simulink model "ModeAdjust"  (R2018b)
settings: Solver=FixedStepDiscrete  StartTime=0.0  StopTime=inf  FixedStep=0.01  RelTol=1e-3
undefined symbols (not defined in the file or in its folder): IfKeSMSbSeatMovBkRclnEnable_Val, IfKeSMSbSeatMovFrwdBkwdEnable_Val, IfKeSMSbSeatMovFtrstEnable_Val, IfKeSMSbSeatMovHdrstFrwdBkwdEnable_Val, IfKeSMSbSeatMovHdUpwdDnwdEnable_Val, IfKeSMSbSeatMovLgrstEnable_Val, IfKeSMSbSeatMovLtwdRtwdEnable_Val, IfVeSMSeStNumConfig, KeSMSbArmscreenMovEnable_Val, KeSMSbSeatMovLgrstExpdEnable_Val, KeSMSuFirstRwStBackPosDelta_Val, KeSMSuFirstRwStBackPosTolr_Val, KeSMSuFirstRwStCushFrntPosDelta_Val, KeSMSuFirstRwStCushFrntPosTolr_Val, KeSMSuFirstRwStCushRePosDelta_Val, KeSMSuFirstRwStCushRePosTolr_Val, KeSMSuFirstRwStFootrestPosDelta_Val, KeSMSuFirstRwStFootrestPosTolr_Val, KeSMSuFirstRwStFwdBkwdPosDelta_Val, KeSMSuFirstRwStFwdBkwdPosTolr_Val, KeSMSuMdMotFinshdTm_Val, KeSMSuMdRetryTm1_Val, KeSMSuModeReqDurgTm_Val, KeSMSuSecRwStArmTochPosDelta_Val, KeSMSuSecRwStArmTochPosTolr_Val, KeSMSuSecRwStBackPosDelta_Val, KeSMSuSecRwStBackPosTolr_Val, KeSMSuSecRwStFtrstUpwdDnwdPosDelta_Val, KeSMSuSecRwStFtrstUpwdDnwdPosTolr_Val, KeSMSuSecRwStFwdBkwdPosDelta_Val, KeSMSuSecRwStFwdBkwdPosTolr_Val, KeSMSuSecRwStHeadrestFwdBkwdPosDelta_Val, KeSMSuSecRwStHeadrestFwdBkwdPosTolr_Val, KeSMSuSecRwStHeadrestUpwdDwnwdPosDelta_Val, KeSMSuSecRwStHeadrestUpwdDwnwdPosTolr_Val, KeSMSuSecRwStLegrestInOutPosDelta_Val, KeSMSuSecRwStLegrestInOutPosTolr_Val, KeSMSuSecRwStLegrestUpwdDwnwdPosDelta_Val, KeSMSuSecRwStLegrestUpwdDwnwdPosTolr_Val, KeSMSuSecRwStLwdRwdPosDelta_Val, KeSMSuSecRwStLwdRwdPosTolr_Val, KeSMSuSecRwStVIPFtrstRefAngle_Val, KeSMSuThirdRwStFwdBkwdPosDelta_Val, KeSMSuThirdRwStFwdBkwdPosTolr_Val, KeSMSuThrdRwCushFoldPosDelta_Val, KeSMSuThrdRwCushFoldPosTolr_Val, KeSMSuThrdRwStBackPosDelta_Val, KeSMSuThrdRwStBackPosTolr_Val, KeSMSw4SLegrstCloseMdSecRwLtStFtrstUpwdDnwdPos_Val, KeSMSw4SLegrstCloseMdSecRwLtStFtrstUpwdDnwdPosMax_Val, KeSMSw4SLegrstCloseMdSecRwLtStFtrstUpwdDnwdPosMin_Val, KeSMSw4SLegrstCloseMdSecRwLtStLgrstOtwdInwdPos_Val, KeSMSw4SLegrstCloseMdSecRwLtStLgrstOtwdInwdPosMax_Val, KeSMSw4SLegrstCloseMdSecRwLtStLgrstOtwdInwdPosMin_Val, KeSMSw4SLegrstCloseMdSecRwLtStLgrstUpwdDnwdPos_Val, KeSMSw4SLegrstCloseMdSecRwLtStLgrstUpwdDnwdPosMax_Val, KeSMSw4SLegrstCloseMdSecRwLtStLgrstUpwdDnwdPosMin_Val, KeSMSw4SLegrstCloseMdSecRwRtStFtrstUpwdDnwdPos_Val, KeSMSw4SLegrstCloseMdSecRwRtStFtrstUpwdDnwdPosMax_Val, KeSMSw4SLegrstCloseMdSecRwRtStFtrstUpwdDnwdPosMin_Val ... (+1138)
libraries: Lib x401
(part 10 of 35)

== system ModeAdjust/ModeAdjustRunnable_sys/ModeAdjust/RecvyR4s ==
  note: Change Request 179276
      | 复位模式头枕上下移动到第一步，第一步直接控制靠背、头枕上下、腿托系统同时运动，
      | 当腿托系统运动完成后进行头枕前后运动
  SecRwLtStsPoss : Inport
  SecRwLtStPossV : Inport  Port=2
  SecRwRtStChldLkRsp_L : Inport  Port=3
  Recovery_Mod_Left : Inport  Port=4
  ModeStCalib : Inport  Port=5
  StConfig : Inport  Port=6
  SecRwLtStsPoss4s : Inport  Port=7
  SecRwLtStPossV4s : Inport  Port=8
  StConfig4s : Inport  Port=9
  isRtRecoveryArrivedAtTargetPos : Inport  Port=10
  Calib_Recovery4sRAdpt : Inport  Port=11
  Enable : EnablePort  StatesWhenEnabling=reset
  Bus Creator1 : BusCreator  Inputs=2
  Bus Selector : BusSelector  OutputSignals=Calib_Drv,Calib_Pass,Calib_2L,Calib_2R,Calib_3L,Calib_3R,Calib_2L4s,Calib_2R4s
  Bus Selector1 : BusSelector  OutputSignals=DrvStConfig,PassStConfig,SecRwLtStConfig,SecRwRtStConfig,ThdRwLtStConfig,ThdRwRtStConfig
  Bus Selector2 : BusSelector  OutputSignals=SecRwLtStConfig,SecRwRtStConfig
  Bus Selector3 : BusSelector  OutputSignals=IfVeSMSuSecRwRtStBkReclnUpwdDnwdPos_Val_read,IfVeSMSuSecRwRtStFrwdBkwdPos_Val_read,IfVeSMSuSecRwRtStHPassStUpwdDnwdPos_Val_read,IfVeSMSuSecRwRtStLgrstUpwdDnwdPos_Val_read,IfVeSMSuSecRwRtStLtwdRtwdPos_Val_read,SecRwRtStArmScrnPos_Val_read
  Bus Selector4 : BusSelector  OutputSignals=IfVeSMSuSecRwRtStBkReclnUpwdDnwdPosV_Val_read,IfVeSMSuSecRwRtStFrwdBkwdPosV_Val_read,IfVeSMSuSecRwRtStHPassStUpwdDnwdPosV_Val_read,IfVeSMSuSecRwRtStLgrstUpwdDnwdPosV_Val_read,IfVeSMSuSecRwRtStLtwdRtwdPosV_Val_read,SecRwRtStArmScrnPosV_Val_read
  Bus Selector5 : BusSelector  OutputSignals=IfVeSMSuSecRwRtStLgrstOtwdInwdPos_Val_read,IfVeSMSuRrRtStFtUpwdDnwdPos_Val_read,IfVeSMSuSecRwRtStHdrstFrwdBkwdPos_Val_read
  Bus Selector6 : BusSelector  OutputSignals=IfVeSMSuSecRwRtStLgrstOtwdInwdPosV_Val_read,IfVeSMSuRrRtStFtUpwdDnwdPosV_Val_read
  Chart : Stateflow chart  TreatAsAtomicUnit=on
  Chart1 : Stateflow chart  TreatAsAtomicUnit=on
  Logical Operator : Logic  Inputs=4  AllPortsSameDT=off  OutDataTypeStr=boolean
  Logical Operator1 : Logic  Operator=NOT  AllPortsSameDT=off  OutDataTypeStr=boolean
  Logical Operator2 : Logic  Inputs=3  AllPortsSameDT=off  OutDataTypeStr=boolean
  Logical Operator3 : Logic  Operator=OR  AllPortsSameDT=off  OutDataTypeStr=boolean
  PA_KeSMSuSecRwStFtrstUpwdDnwdPosDelta_Val : Constant  Value=KeSMSuSecRwStFtrstUpwdDnwdPosDelta_Val
  PA_KeSMSuSecRwStLegrestInOutPosDelta_Val : Constant  Value=KeSMSuSecRwStLegrestInOutPosDelta_Val
  PA_KeSMSw4SSecRwRtStLgrstOtwdInwdClosePos1_Val : Constant  Value=KeSMSw4SSecRwRtStLgrstOtwdInwdClosePos1_Val
  PA_KeSMSw4SSecRwRtStLgrstUpwdDnwdClosePos1_Val : Constant  Value=KeSMSw4SSecRwRtStLgrstUpwdDnwdClosePos1_Val
  PA_KeSMSw4SSecRwRtStLgrstUpwdDnwdClosePos2_Val : Constant  Value=KeSMSw4SSecRwRtStLgrstUpwdDnwdClosePos2_Val
  R2Lt : Subsystem
  VIP_TrigJudg : Lib/VIP_TrigJudg  SystemSampleTime=-1
  R2Lt_TrgtPoss : Outport  VectorParamsAs1DForOutWhenUnconnected=on
  IfVeSMSuSecRwLtStRclCmdSrv_Val_writeRec : Outport  Port=2
  isAcsMdFeedBackNew_LyL : Outport  Port=3
  R2Lt_TrgtPoss_2 : Outport  Port=4  VectorParamsAs1DForOutWhenUnconnected=on
  wires:
  R2Lt/6(lgrstFtUpwd_ini) -> [lgrstStep3_ini]
  R2Lt/7(lgrstOtwd_ini) -> [lgrstStep1_ini]
  R2Lt/5(lgrstUpwd_ini) -> [lgrstStep2_ini]
  R2Lt/9(lgrstStep2_done) -> [lgrstStep3_done]
  R2Lt/10(lgrstStep3_done) -> [lgrstStep1_done]
  R2Lt/8(lgrstStep1_done) -> [lgrstStep2_done]
  [KeSMSuSecRwStFtrstUpwdDnwdPosDelta_Val] -> Chart/15(FtposDelta)
  PA_KeSMSuSecRwStFtrstUpwdDnwdPosDelta_Val/1 -> [KeSMSuSecRwStFtrstUpwdDnwdPosDelta_Val]
  [StepEn_LgrstStep2] -> R2Lt/11(StepEn_LgrstStep1)
  [StepEn_LgrstStep3] -> R2Lt/12(StepEn_LgrstStep2)
  [StepEn_LgrstStep1] -> R2Lt/13(StepEn_LgrstStep3)
  [SecRwLtStLgrstOtwdInwdPos] -> Chart/4(Otpos)
  [RrLtStFtUpwdDnwdPos] -> Chart/5(Ftpos)
  [CloseOtwdPos1] -> Chart/8(closeOtpos1)
  [CloseDnwdPos1] -> Chart/6(closedownpos1)
  [CloseDnwdPos2] -> Chart/7(closedownpos2)
  PA_KeSMSw4SSecRwRtStLgrstUpwdDnwdClosePos1_Val/1 -> [CloseDnwdPos1]
  PA_KeSMSw4SSecRwRtStLgrstUpwdDnwdClosePos2_Val/1 -> [CloseDnwdPos2]
  PA_KeSMSw4SSecRwRtStLgrstOtwdInwdClosePos1_Val/1 -> [CloseOtwdPos1]
  [lgrstStep3_done] -> Chart/11(Step3done)
  R2Lt/11(R2Lt_TrgtPoss_2) -> R2Lt_TrgtPoss_2/1
  Chart/4(StepEn_LgrstStep3) -> [StepEn_LgrstStep3]
  Chart/3(StepEn_LgrstStep2) -> [StepEn_LgrstStep2]
  Chart/2(StepEn_LgrstStep1) -> [StepEn_LgrstStep1]
  [lgrstStep2_done] -> Chart/10(Step2done)
  [lgrstStep3_ini] -> Chart/14(Step3_ini)
  [lgrstStep2_ini] -> Chart/13(Step2_ini)
  [lgrstStep1_ini] -> Chart/12(Step1_ini)
  [lgrstStep1_done] -> Chart/9(Step1done)
  [SecRwLtStLgrstUpwdDnwdPos] -> Chart/3(downpos)
  Bus Selector5/2 -> [RrLtStFtUpwdDnwdPos]  "<IfVeSMSuRrRtStFtUpwdDnwdPos_Val_read>"
  Bus Selector5/1 -> [SecRwLtStLgrstOtwdInwdPos]  "<IfVeSMSuSecRwRtStLgrstOtwdInwdPos_Val_read>"
  [PosV4s] -> Bus Selector6/1
  Bus Selector6/2 -> [RrLtStFtUpwdDnwdPosV]  "<IfVeSMSuRrRtStFtUpwdDnwdPosV_Val_read>"
  [Pos4s] -> Bus Selector5/1
  Bus Selector6/1 -> [SecRwLtStLgrstOtwdInwdPosV]  "<IfVeSMSuSecRwRtStLgrstOtwdInwdPosV_Val_read>"
  Bus Selector4/1 -> [SecRwLtStBkReclnUpwdDnwdPosV]  "<IfVeSMSuSecRwRtStBkReclnUpwdDnwdPosV_Val_read>"
  Bus Selector4/3 -> [SecRwLtStHPassStUpwdDnwdPosV]  "<IfVeSMSuSecRwRtStHPassStUpwdDnwdPosV_Val_read>"
  Bus Selector3/5 -> [SecRwLtStLtwdRtwdPos]  "<IfVeSMSuSecRwRtStLtwdRtwdPos_Val_read>"
  [Pos] -> Bus Selector3/1
  Bus Selector3/3 -> [SecRwLtStHPassStUpwdDnwdPos]  "<IfVeSMSuSecRwRtStHPassStUpwdDnwdPos_Val_read>"
  Bus Selector4/4 -> [SecRwLtStLgrstUpwdDnwdPosV]  "<IfVeSMSuSecRwRtStLgrstUpwdDnwdPosV_Val_read>"
  Bus Selector4/2 -> [SecRwLtStFrwdBkwdPosV]  "<IfVeSMSuSecRwRtStFrwdBkwdPosV_Val_read>"
  Bus Selector3/2 -> [SecRwLtStFrwdBkwdPos]  "<IfVeSMSuSecRwRtStFrwdBkwdPos_Val_read>"
  Bus Selector3/1 -> [SecRwLtStBkReclnUpwdDnwdPos]  "<IfVeSMSuSecRwRtStBkReclnUpwdDnwdPos_Val_read>"
  Bus Selector3/4 -> [SecRwLtStLgrstUpwdDnwdPos]  "<IfVeSMSuSecRwRtStLgrstUpwdDnwdPos_Val_read>"
  Bus Selector4/5 -> [SecRwLtStLtwdRtwdPosV]  "<IfVeSMSuSecRwRtStLtwdRtwdPosV_Val_read>"
  Bus Selector3/6 -> [R2LtStArmScrnPos]  "<SecRwRtStArmScrnPos_Val_read>"
  Bus Selector4/6 -> [R2LtStArmScrnPosV]  "<SecRwRtStArmScrnPosV_Val_read>"
  [PosV] -> Bus Selector4/1
  [SecRwLtStConfig4s] -> R2Lt/10(StConfig4s)
  Bus Selector2/2 -> [SecRwRtStConfig4s]  "<SecRwRtStConfig>"
  Bus Selector2/1 -> [SecRwLtStConfig4s]  "<SecRwLtStConfig>"
  StConfig4s/1 -> Bus Selector2/1
  SecRwLtStPossV4s/1 -> R2Lt/9(SecRwLtStPossV4s), [PosV4s]
  SecRwLtStsPoss4s/1 -> [Pos4s], R2Lt/8(SecRwLtStsPoss4s)
  Bus Selector/7 -> [ModeStCalib_2L4s]  "<Calib_2L4s>"
  Bus Selector/8 -> [ModeStCalib_2R4s]  "<Calib_2R4s>"
  [SecRwLtStConfig] -> R2Lt/7(StConfig)
  Bus Selector1/5 -> [ThdRwLtStConfig]  "<ThdRwLtStConfig>"
  Bus Selector1/2 -> [PassStConfig]  "<PassStConfig>"
  StConfig/1 -> Bus Selector1/1
  Bus Selector1/4 -> [SecRwRtStConfig]  "<SecRwRtStConfig>"
  Bus Selector1/3 -> [SecRwLtStConfig]  "<SecRwLtStConfig>"
  Bus Selector1/1 -> [DrvStConfig]  "<DrvStConfig>"
  Bus Selector1/6 -> [ThdRwRtStConfig]  "<ThdRwRtStConfig>"
  [Ly_L_DoneFailed] -> Bus Creator1/2  "isRfRecoveryDoneFailed"
  [Ly_L_DoneOK] -> Bus Creator1/1  "isRfRecoveryDoneOK"
  Bus Creator1/1 -> isAcsMdFeedBackNew_LyL/1
  [Recovery_Mod_Left] -> VIP_TrigJudg/1
  [ModeStCalib_2R4s] -> R2Lt/6(ModeStCalib_2L)
  ModeStCalib/1 -> Bus Selector/1
  Bus Selector/4 -> [ModeStCalib_2R]  "<Calib_2R>"
  Bus Selector/6 -> [ModeStCalib_3R]  "<Calib_3R>"
  Bus Selector/1 -> [ModeStCalib_Drv]  "<Calib_Drv>"
  Bus Selector/3 -> [ModeStCalib_2L]  "<Calib_2L>"
  Bus Selector/5 -> [ModeStCalib_3L]  "<Calib_3L>"
  Bus Selector/2 -> [ModeStCalib_Pass]  "<Calib_Pass>"
  Chart1/1(IfVeSMSuSecRwLtStRclCmdSrv_Val_write) -> IfVeSMSuSecRwLtStRclCmdSrv_Val_writeRec/1  "IfVeSMSuSecRwLtStRclCmdSrv_Val_write"
  Chart1/3(Md_L_DoneFailed) -> [Ly_L_DoneFailed]
  Chart1/2(Md_L_DoneOk) -> [Ly_L_DoneOK]
  [Recv_L_DoneFailed] -> Chart1/4(Md_L_DoneFailedRaw)
  [Recv_L_DoneOK] -> Chart1/3(Md_L_DoneOkRaw)
  Chart/1(R2Lt_En) -> [Step1_En]
  [R2LtST_BkHd_done] -> Chart/2(R2Lt_done)
  [R2LtST_BkHd_ini] -> Chart/1(R2Lt_ini)
  R2Lt/2(R2Lt_BkHd_done) -> [R2LtST_BkHd_done]
  SecRwRtStChldLkRsp_L/1 -> R2Lt/5(SecRwRtStChldLkRsp_L)
  SecRwLtStPossV/1 -> [PosV], R2Lt/4(SecRwLtStPossV)
  SecRwLtStsPoss/1 -> [Pos], R2Lt/3(SecRwLtStsPoss)
  R2Lt/3(R2Lt_TrgtPoss) -> R2Lt_TrgtPoss/1
  [EZE_TrigL] -> R2Lt/1(Mode_Trig)
  VIP_TrigJudg/1 -> [EZE_TrigL]
  [Step1_En] -> R2Lt/2(Step1En)
  R2Lt/1(R2Lt_BkHd_Ini) -> [R2LtST_BkHd_ini]
  Logical Operator/1 -> Chart1/1(Left_Done)
  Recovery_Mod_Left/1 -> [Recovery_Mod_Left]
  [IfVeSMSuSecRwLtStRclCmdSrv_Val_writeRaw] -> Chart1/2(IfVeSMSuSecRwLtStRclCmdSrv_Val_writeRaw)
  R2Lt/4(IfVeSMSuSecRwLtStRclCmdSrv_Val_writeRaw) -> [IfVeSMSuSecRwLtStRclCmdSrv_Val_writeRaw]
  Logical Operator1/1 -> [Recv_L_DoneFailed]
  isRtRecoveryArrivedAtTargetPos/1 -> [Recv_L_DoneOK], Logical Operator1/1
  Chart/5(HdUp_En) -> [HdUp_En]
  Chart/6(HdFwd_En) -> [HdFwd_En]
  [HdUp_Done] -> Chart/17(HdUp_Done)
  [HFwd_Done] -> Chart/16(HdFwd_Done)
  Bus Selector5/3 -> [SecRwLtStHdrstFrwdBkwdPos]  "<IfVeSMSuSecRwRtStHdrstFrwdBkwdPos_Val_read>"
  R2Lt/14(R2Lt_HdFwd_Ini) -> [HFwd_ini]
  R2Lt/12(R2Lt_HdUp_Ini) -> [HdUp_ini]
  R2Lt/15(R2Lt_HdFwd_Done) -> [HFwd_Done]
  R2Lt/13(R2Lt_HdUp_Done) -> [HdUp_Done]
  [HdUp_En] -> R2Lt/14(HdUp_En)
  [HdFwd_En] -> R2Lt/15(HdFwd_En)
  PA_KeSMSuSecRwStLegrestInOutPosDelta_Val/1 -> [KeSMSuSecRwStLegrestInOutPosDelta_Val]
  [KeSMSuSecRwStLegrestInOutPosDelta_Val] -> Chart/18(OtposDelta)
  Chart/7(failflg) -> [failflg]
  [lgrstStep1_done] -> Logical Operator2/1
  [lgrstStep2_done] -> Logical Operator2/2
  [lgrstStep3_done] -> Logical Operator2/3
  Logical Operator2/1 -> Logical Operator3/2
  [failflg] -> Logical Operator3/1
  Logical Operator3/1 -> Logical Operator/1
  [HdUp_Done] -> Logical Operator/4
  [HFwd_Done] -> Logical Operator/3
  [R2LtST_BkHd_done] -> Logical Operator/2
  [HdUp_ini] -> Chart/19(HdUp_ini)
  [HFwd_ini] -> Chart/20(HFwd_ini)
  Calib_Recovery4sRAdpt/1 -> R2Lt/16(Calib_Recovery4sRAdpt)

== system ModeAdjust/ModeAdjustRunnable_sys/ModeAdjust/SeatOccupyCheck ==
  IfVeSMSeNotThdRwCtStOccStatMSMSrc_Val_read : Inport
  IfVeSMSeNotThdRwLtStOccStatMSMSrc_Val_read : Inport  Port=2
  IfVeSMSeNotThdRwRtStOccStatMSMSrc_Val_read : Inport  Port=3
  StNumConfig : Inport  Port=4
  Bus Creator : BusCreator  Inputs=3
  Bus Creator1 : BusCreator  Inputs=3
  Bus Creator2 : BusCreator  Inputs=3
  Bus Selector : BusSelector  OutputSignals=LtStOccStat,CtStOccStat,RtStOccStat
  Constant{,1..3} (4 alike) : Constant  Value=SeatOccupiedSts1.SeatOccupiedSts_Empty  OutDataTypeStr=Enum:SeatOccupiedSts1
  Multiport Switch4 : MultiPortSwitch  DataPortOrder=Specify indices  DataPortIndices={IfVeSMSeStNumConfig.SeatNum4Config,IfVeSMSeStNumConfig.SeatNum6Config,IfVeSMSeStNumConfig.SeatNum7Config,IfVeSMSeStNumConfig.SeatNum4PConfig}  DataPortForDefault=Additional data port  DiagnosticForDefault=None
  SeatOccupiedStat : Lib/SeatOccupiedStat  SystemSampleTime=-1
  SeatOccupiedStat1 : Lib/SeatOccupiedStat  SystemSampleTime=-1
  SeatOccupiedStat2 : Lib/SeatOccupiedStat  SystemSampleTime=-1
  isR3LfSeatOccupied : Outport
  isR3MidSeatOccupied : Outport  Port=2
  isR3RtSeatOccupied : Outport  Port=3
  wires:
  SeatOccupiedStat/1 -> isR3LfSeatOccupied/1  "isR3LfSeatOccupied"
  SeatOccupiedStat1/1 -> isR3MidSeatOccupied/1  "isR3MidSeatOccupied"
  SeatOccupiedStat2/1 -> isR3RtSeatOccupied/1  "isR3RtSeatOccupied"
  StNumConfig/1 -> Multiport Switch4/1
  IfVeSMSeNotThdRwCtStOccStatMSMSrc_Val_read/1 -> Bus Creator/2  "CtStOccStat"
  Bus Creator/1 -> Multiport Switch4/6, Multiport Switch4/4
  Multiport Switch4/1 -> Bus Selector/1
  Constant2/1 -> Bus Creator1/3  "RtStOccStat"
  Constant/1 -> Bus Creator1/1  "LtStOccStat"
  Bus Creator1/1 -> Multiport Switch4/2, Multiport Switch4/5
  Constant1/1 -> Bus Creator1/2  "CtStOccStat"
  Constant3/1 -> Bus Creator2/2  "CtStOccStat"
  Bus Creator2/1 -> Multiport Switch4/3
  IfVeSMSeNotThdRwLtStOccStatMSMSrc_Val_read/1 -> Bus Creator/1, Bus Creator2/1  "LtStOccStat"
  IfVeSMSeNotThdRwRtStOccStatMSMSrc_Val_read/1 -> Bus Creator2/3, Bus Creator/3  "RtStOccStat"
  Bus Selector/1 -> SeatOccupiedStat/1  "<LtStOccStat>"
  Bus Selector/2 -> SeatOccupiedStat1/1  "<CtStOccStat>"
  Bus Selector/3 -> SeatOccupiedStat2/1  "<RtStOccStat>"

== system ModeAdjust/ModeAdjustRunnable_sys/ModeAdjust/SecRowSeatOccupyCheck ==
  IfVeSMSeNotSecRowLeSeaOccStat_Val_read : Inport
  IfVeSMSeNotSecRowRtSeaOccStat_Val_read : Inport  Port=2
  SeatOccupiedStat : Lib/SeatOccupiedStat  SystemSampleTime=-1
  SeatOccupiedStat1 : Lib/SeatOccupiedStat  SystemSampleTime=-1
  isSecRowLtSeatOccupied : Outport  VectorParamsAs1DForOutWhenUnconnected=on
  isSecRowRtSeatOccupied : Outport  Port=2  VectorParamsAs1DForOutWhenUnconnected=on
  wires:
  IfVeSMSeNotSecRowLeSeaOccStat_Val_read/1 -> SeatOccupiedStat/1
  IfVeSMSeNotSecRowRtSeaOccStat_Val_read/1 -> SeatOccupiedStat1/1
  SeatOccupiedStat/1 -> isSecRowLtSeatOccupied/1  "isSecRowLtSeatOccupied"
  SeatOccupiedStat1/1 -> isSecRowRtSeatOccupied/1  "isSecRowRtSeatOccupied"

== system ModeAdjust/ModeAdjustRunnable_sys/ModeAdjust/Subsystem ==
  StNumConfig : Inport
  Logical Operator1 : Logic  Operator=OR  AllPortsSameDT=off  OutDataTypeStr=boolean
  Logical Operator9 : Logic  Operator=OR  AllPortsSameDT=off  OutDataTypeStr=boolean
  PA_KeSMSwDltTrgtPos_Val1 : Constant  Value=IfVeSMSeStNumConfig.SeatNum6Config  OutDataTypeStr=Enum:IfVeSMSeStNumConfig
  PA_KeSMSwDltTrgtPos_Val10 : Constant  Value=IfVeSMSeStNumConfig.SeatNum7Config  OutDataTypeStr=Enum:IfVeSMSeStNumConfig
  PA_KeSMSwDltTrgtPos_Val2 : Constant  Value=IfVeSMSeStNumConfig.SeatNum4Config  OutDataTypeStr=Enum:IfVeSMSeStNumConfig
  PA_KeSMSwDltTrgtPos_Val3 : Constant  Value=IfVeSMSeStNumConfig.SeatNum4PConfig  OutDataTypeStr=Enum:IfVeSMSeStNumConfig
  Relational Operator{1..3,10} (4 alike) : RelationalOperator  Operator===  OutDataTypeStr=boolean  RndMeth=Simplest
  is6s7s : Outport
  is4s : Outport  Port=2
  is6s : Outport  Port=3
  is7s : Outport  Port=4
  wires:
  Relational Operator1/1 -> is6s/1, Logical Operator9/1  "is6s"
  Logical Operator9/1 -> is6s7s/1  "is6s7s"
  [StNumConfig] -> Relational Operator1/1
  [StNumConfig] -> Relational Operator10/1
  PA_KeSMSwDltTrgtPos_Val1/1 -> Relational Operator1/2
  Relational Operator10/1 -> is7s/1, Logical Operator9/2  "is7s"
  PA_KeSMSwDltTrgtPos_Val10/1 -> Relational Operator10/2
  StNumConfig/1 -> [StNumConfig]
  [StNumConfig] -> Relational Operator2/1
  PA_KeSMSwDltTrgtPos_Val2/1 -> Relational Operator2/2
  [StNumConfig] -> Relational Operator3/1
  PA_KeSMSwDltTrgtPos_Val3/1 -> Relational Operator3/2
  Relational Operator2/1 -> Logical Operator1/1
  Relational Operator3/1 -> Logical Operator1/2
  Logical Operator1/1 -> is4s/1  "is4s"

== system ModeAdjust/ModeAdjustRunnable_sys/ModeAdjust/VIPL ==
  SecRwLtStsPoss : Inport
  SecRwLtStPossV : Inport  Port=2
  ThdRwLtStPoss : Inport  Port=3
  ThdRwLtStPossV : Inport  Port=4
  SecRwRtStChldLkRsp_L : Inport  Port=5
  isR3MidSeatOccupied : Inport  Port=6
  isR3LfSeatOccupied : Inport  Port=7
  VIP_Mod_Left : Inport  Port=8
  ModeStCalib : Inport  Port=9
  StConfig : Inport  Port=10
  DrvCurPos : Inport  Port=11
  DrvCurPosV : Inport  Port=12
  isLfVipArrivedAtTargetPos : Inport  Port=13
  Drv_FtUpwdDnwdPosTrgt : Inport  Port=14
  Enable : EnablePort  StatesWhenEnabling=reset
  Bus Creator1 : BusCreator  Inputs=2
  Bus Selector : BusSelector  OutputSignals=Calib_Drv,Calib_Pass,Calib_2L,Calib_2R,Calib_3L,Calib_3R
  Bus Selector1 : BusSelector  OutputSignals=DrvStConfig,PassStConfig,SecRwLtStConfig,SecRwRtStConfig,ThdRwLtStConfig,ThdRwRtStConfig
  Chart1 : Stateflow chart  TreatAsAtomicUnit=on
  Chart2 : Stateflow chart  TreatAsAtomicUnit=on
  Drv : Subsystem
  Logical Operator{,5,9,12} (4 alike) : Logic  Inputs=3  AllPortsSameDT=off  OutDataTypeStr=boolean
  Logical Operator{1,11,14..15} (4 alike) : Logic  AllPortsSameDT=off  OutDataTypeStr=boolean
  Logical Operator{4,6..7,13} (4 alike) : Logic  Operator=OR  AllPortsSameDT=off  OutDataTypeStr=boolean
  Logical Operator2 : Logic  Operator=NOT  AllPortsSameDT=off  OutDataTypeStr=boolean
  R2Lt : Subsystem
  R3Lt : Subsystem
  Terminator3 : Terminator
  Unit Delay1 : UnitDelay  SampleTime=-1
  Unit Delay3 : UnitDelay  SampleTime=-1
  Unit Delay4 : UnitDelay  SampleTime=-1
  VIP_TrigJudg : Lib/VIP_TrigJudg  SystemSampleTime=-1
  R2Lt_TrgtPoss : Outport  VectorParamsAs1DForOutWhenUnconnected=on
  R3Lt_TrgtPoss : Outport  Port=2  VectorParamsAs1DForOutWhenUnconnected=on
  IfVeSMSbThdRwLtStRclCmdSrv_Val_writeVIP : Outport  Port=3
  IfVeSMSuSecRwLtStRclCmdSrv_Val_writeVIP : Outport  Port=4
  isAcsMdFeedBackNew_VIPL : Outport  Port=5
  VIPLDone : Outport  Port=6
  DrvStTrgtPoss : Outport  Port=7  VectorParamsAs1DForOutWhenUnconnected=on
  IfVeSMSuDrvStRclCmdSrv_Val_write : Outport  Port=8
  R2Lt_SpdCtrl : Outport  Port=9  VectorParamsAs1DForOutWhenUnconnected=on
  R3Lt_SpdCtrl : Outport  Port=10  VectorParamsAs1DForOutWhenUnconnected=on
  wires:
  isR3MidSeatOccupied/1 -> Logical Operator4/1
  SecRwRtStChldLkRsp_L/1 -> [SecRwRtStChldLkRsp_L], R2Lt/7(SecRwRtStChldLkRsp_L)
  ThdRwLtStPossV/1 -> R3Lt/5(ThdRwLtStPossV)
  ThdRwLtStPoss/1 -> R3Lt/4(ThdRwLtStPoss)
  SecRwLtStPossV/1 -> R2Lt/6(SecRwLtStPossV)
  SecRwLtStsPoss/1 -> R2Lt/5(SecRwLtStsPoss)
  [EZE_TrigL] -> R3Lt/1(Mode_Trig)
  R3Lt/4(R3Lt_TrgtPoss) -> R3Lt_TrgtPoss/1
  R2Lt/7(R2Lt_TrgtPoss) -> R2Lt_TrgtPoss/1
  [EZE_TrigL] -> R2Lt/1(Mode_Trig)
  [IfVeSMSbThdRwLtStRclCmdSrv_Val_writeRaw] -> Chart1/2(IfVeSMSbThdRwLtStRclCmdSrv_Val_writeRaw)
  R3Lt/3(IfVeSMSbThdRwLtStRclCmdSrv_Val_writeRaw) -> [IfVeSMSbThdRwLtStRclCmdSrv_Val_writeRaw]
  R2Lt/6(R2Lt_Step2_done) -> [R2LtST_Step2_done]  "VIPL_R2LtST_Step2_done"
  R2Lt/5(R2Lt_Step1_done) -> [R2LtST_Step1_done]  "VIPL_R2LtST_Step1_done"
  R2Lt/4(R2Lt_Step2_Ini) -> [R2LtST_Step2_ini]
  R2Lt/1(R2Lt_Step1_Ini) -> [R2LtST_Step1_ini]
  R3Lt/1(R3Lt_Step1_ini) -> [R3Lt_Step1_ini]
  Logical Operator4/1 -> [Occupied]
  isR3LfSeatOccupied/1 -> Logical Operator4/2
  VIP_TrigJudg/1 -> [EZE_TrigL]
  R3Lt/2(R3Lt_Step1done) -> [R3Lt_Step1_done]  "VIPL_R3Lt_Step1_done"
  Chart2/1(L_R3Step1) -> [L_R3Step1]
  Chart2/2(L_R2Step1) -> [L_R2Step1]
  Chart2/3(L_R2Step2) -> [L_R2Step2]
  Chart2/4(L_R2Step3) -> [L_R2Step3]
  [R3Lt_Step1_ini] -> [L_R3_ini]
  [L_R3Step1] -> R3Lt/2(Step1En)
  [L_R2Step1] -> R2Lt/2(Step1En)
  [L_R2Step2] -> R2Lt/3(Step2En)
  [L_R2Step3] -> R2Lt/4(Step3En)
  R2Lt/8(R2Lt_Step3_Ini) -> [R2LtST_Step3_ini]
  R2Lt/9(R2Lt_Step3_done) -> [R2LtST_Step3_done]  "VIPL_R2LtST_Step3_done"
  [R3Lt_Step1_ini] -> Chart2/1(L_R3Step1_ini)
  [R2LtST_Step1_ini] -> Chart2/2(L_R2Step1_ini)
  [R2LtST_Step2_ini] -> Chart2/3(L_R2Step2_ini)
  [R2LtST_Step3_ini] -> Chart2/4(L_R2Step3_ini)
  R2Lt/2(ini_ReclnOverUp) -> [L_ini_ReclnOverUp]
  [L_ini_ReclnOverUp] -> Chart2/5(L_PosOvrup)
  R2Lt/3(ini_ReclnOverDwn) -> Terminator3/1
  [R2LtST_Step1_done] -> Chart2/7(L_R2Step1done)
  [R2LtST_Step2_done] -> Chart2/8(L_R2Step2done)
  [R3Lt_Step1_done] -> Chart2/6(L_R3Step1done)
  [R2LtST_Step1_ini] -> Logical Operator5/1
  [R2LtST_Step2_ini] -> Logical Operator5/2
  [R2LtST_Step3_ini] -> Logical Operator5/3
  Logical Operator5/1 -> [L_R2_ini]
  VIP_Mod_Left/1 -> [VIP_Left]
  [IfVeSMSuSecRwLtStRclCmdSrv_Val_writeRaw] -> Chart1/3(IfVeSMSuSecRwLtStRclCmdSrv_Val_writeRaw)
  R2Lt/10(IfVeSMSuSecRwLtStRclCmdSrv_Val_writeRaw) -> [IfVeSMSuSecRwLtStRclCmdSrv_Val_writeRaw]
  [VIP_Left] -> R2Lt/8(VIP_Left)
  [Md_L_MvDoneOK] -> Chart1/4(Md_L_DoneOkRaw)
  [Md_L_MvDoneFailed] -> Chart1/5(Md_L_DoneFailedRaw)
  Chart1/3(Md_L_DoneOk) -> [VIP_L_DoneOK]
  Chart1/4(Md_L_DoneFailed) -> [VIP_L_DoneFailed]
  Chart1/1(IfVeSMSbThdRwLtStRclCmdSrv_Val_write) -> IfVeSMSbThdRwLtStRclCmdSrv_Val_writeVIP/1  "IfVeSMSbThdRwLtStRclCmdSrv_Val_write"
  Chart1/2(IfVeSMSuSecRwLtStRclCmdSrv_Val_write) -> IfVeSMSuSecRwLtStRclCmdSrv_Val_writeVIP/1  "IfVeSMSuSecRwLtStRclCmdSrv_Val_write"
  R2Lt/11(R2Lt_All_done) -> [R2LtST_All_done]
  R3Lt/5(R3Lt_All_done) -> [R3Lt_All_done]
  Bus Selector/2 -> [ModeStCalib_Pass]  "<Calib_Pass>"
  Bus Selector/5 -> [ModeStCalib_3L]  "<Calib_3L>"
  Bus Selector/3 -> [ModeStCalib_2L]  "<Calib_2L>"
  Bus Selector/1 -> [ModeStCalib_Drv]  "<Calib_Drv>"
  Bus Selector/6 -> [ModeStCalib_3R]  "<Calib_3R>"
  Bus Selector/4 -> [ModeStCalib_2R]  "<Calib_2R>"
  ModeStCalib/1 -> Bus Selector/1
  [ModeStCalib_2L] -> R2Lt/9(ModeStCalib_2L)
  [ModeStCalib_3L] -> R3Lt/6(ModeStCalib_3L)
  [VIP_Left] -> VIP_TrigJudg/1
  Bus Creator1/1 -> isAcsMdFeedBackNew_VIPL/1
  [VIP_L_DoneOK] -> Bus Creator1/1  "isLfVipDoneOK"
  [VIP_L_DoneFailed] -> Bus Creator1/2  "isLfVipDoneFailed"
  Bus Selector1/6 -> [ThdRwRtStConfig]  "<ThdRwRtStConfig>"
  Bus Selector1/1 -> [DrvStConfig]  "<DrvStConfig>"
  Bus Selector1/3 -> [SecRwLtStConfig]  "<SecRwLtStConfig>"
  Bus Selector1/4 -> [SecRwRtStConfig]  "<SecRwRtStConfig>"
  StConfig/1 -> Bus Selector1/1
  Bus Selector1/2 -> [PassStConfig]  "<PassStConfig>"
  Bus Selector1/5 -> [ThdRwLtStConfig]  "<ThdRwLtStConfig>"
  [SecRwLtStConfig] -> R2Lt/10(StConfig)
  [ThdRwLtStConfig] -> R3Lt/7(StConfig)
  Logical Operator12/1 -> VIPLDone/1, Chart1/1(LeftDone)
  [Occupied] -> R3Lt/3(isSeatOccupied)
  [Occupied] -> R2Lt/11(isSeatOccupied)
  [SecRwRtStChldLkRsp_L] -> R3Lt/8(SecRwRtStChldLkRsp_L)
  [R2LtST_Step1_done] -> Logical Operator/2
  [R2LtST_Step2_done] -> Logical Operator/3
  [R3Lt_Step1_done] -> Logical Operator/1
  Logical Operator/1 -> Unit Delay1/1
  [Stage1_done] -> Chart2/9(Stage1_done)
  [Stage2_done] -> Chart2/10(Stage2_done)
  Drv/2(DrvSt_Step1_done) -> [DrvST_Step1_done]  "VIPL_DrvST_Step1_done"
  [L_R1Step1] -> Drv/2(Step1En)
  Drv/1(DrvSt_Step1_ini) -> [DrvST_Step1_ini]
  [ModeStCalib_Drv] -> Drv/5(ModeStCalib_Drv)
  DrvCurPos/1 -> Drv/3(DrvCurPos)
  Drv/3(Recv_DrvStTrgtPoss) -> DrvStTrgtPoss/1
  DrvCurPosV/1 -> Drv/4(DrvCurPosV)
  [DrvStConfig] -> Drv/6(StConfig)
  [EZE_TrigL] -> Drv/1(Mode_Trig)
  Chart2/5(L_R1Step1) -> [L_R1Step1]
  [DrvST_Step1_ini] -> Chart2/11(L_R1Step1_ini)
  Drv/4(IfVeSMSuDrvStRclCmdSrv_Val_writeRaw) -> [IfVeSMSuDrvStRclCmdSrv_Val_writeRaw]
  [IfVeSMSuDrvStRclCmdSrv_Val_writeRaw] -> Chart1/6(IfVeSMSuDrvStRclCmdSrv_Val_writeRaw)
  Chart1/5(IfVeSMSuDrvStRclCmdSrv_Val_write) -> IfVeSMSuDrvStRclCmdSrv_Val_write/1
  [Stage1_done] -> Unit Delay3/1
  [DrvST_Step1_done] -> Logical Operator1/1
  Logical Operator6/1 -> [Stage2_done]
  Logical Operator1/1 -> Logical Operator6/2
  Logical Operator7/1 -> [Stage1_done]
  Unit Delay1/1 -> Logical Operator7/2
  [R2LtST_Step1_ini] -> Logical Operator9/1
  [R2LtST_Step2_ini] -> Logical Operator9/2
  [L_R3_ini] -> Logical Operator9/3
  Logical Operator9/1 -> Logical Operator7/1
  [R2LtST_Step3_done] -> Logical Operator11/2
  Logical Operator11/1 -> Logical Operator13/2
  Logical Operator13/1 -> [Stage3_done]
  [Stage2_done] -> Unit Delay4/1
  [Stage1_done] -> Logical Operator12/1
  [Stage2_done] -> Logical Operator12/2
  [Stage3_done] -> Logical Operator12/3
  Unit Delay3/1 -> Logical Operator1/2
  Unit Delay4/1 -> Logical Operator11/1
  Logical Operator14/1 -> Logical Operator6/1
  [DrvST_Step1_ini] -> Logical Operator14/1
  [Stage1_done] -> Logical Operator14/2
  Logical Operator15/1 -> Logical Operator13/1
  [R2LtST_Step3_ini] -> Logical Operator15/1
  [Stage2_done] -> Logical Operator15/2
  [Stage3_done] -> Chart2/12(Stage3_done)
  [SecRwRtStChldLkRsp_L] -> Drv/7(SecRwRtStChldLkRsp_L)
  [Occupied] -> Drv/8(isSeatOccupied)
  Logical Operator2/1 -> [Md_L_MvDoneFailed]
  isLfVipArrivedAtTargetPos/1 -> [Md_L_MvDoneOK], Logical Operator2/1
  Drv_FtUpwdDnwdPosTrgt/1 -> Drv/9(Drv_FtUpwdDnwdPosTrgt)
  R2Lt/12(R2Lt_SpdCtrl) -> R2Lt_SpdCtrl/1
  R3Lt/6(R3Lt_SpdCtrl) -> R3Lt_SpdCtrl/1

== system ModeAdjust/ModeAdjustRunnable_sys/ModeAdjust/VIPL4s ==
  SecRwLtStsPoss : Inport
  SecRwLtStPossV : Inport  Port=2
  SecRwRtStChldLkRsp_L : Inport  Port=3
  Recovery_Mod_Left : Inport  Port=4
  ModeStCalib : Inport  Port=5
  StConfig : Inport  Port=6
  SecRwLtStsPoss4s : Inport  Port=7
  SecRwLtStPossV4s : Inport  Port=8
  StConfig4s : Inport  Port=9
  isLfVipArrivedAtTargetPos : Inport  Port=10
  Calib_VIP4sLAdpt : Inport  Port=11
  Enable : EnablePort  StatesWhenEnabling=reset
  Bus Creator1 : BusCreator  Inputs=2
  Bus Selector : BusSelector  OutputSignals=Calib_Drv,Calib_Pass,Calib_2L,Calib_2R,Calib_3L,Calib_3R,Calib_2L4s,Calib_2R4s
  Bus Selector1 : BusSelector  OutputSignals=DrvStConfig,PassStConfig,SecRwLtStConfig,SecRwRtStConfig,ThdRwLtStConfig,ThdRwRtStConfig
  Bus Selector2 : BusSelector  OutputSignals=SecRwLtStConfig,SecRwRtStConfig
  Bus Selector3 : BusSelector  OutputSignals=IfVeSMSuSecRwLtStBkReclnUpwdDnwdPos_Val_read,IfVeSMSuSecRwLtStFrwdBkwdPos_Val_read,IfVeSMSuSecRwLtStHPassStUpwdDnwdPos_Val_read,IfVeSMSuSecRwLtStLgrstUpwdDnwdPos_Val_read,IfVeSMSuSecRwLtStLtwdRtwdPos_Val_read,IfVeSMSuSecRwLtStArmScrnPos_Val_read
  Bus Selector4 : BusSelector  OutputSignals=IfVeSMSuSecRwLtStBkReclnUpwdDnwdPosV_Val_read,IfVeSMSuSecRwLtStFrwdBkwdPosV_Val_read,IfVeSMSuSecRwLtStHPassStUpwdDnwdPosV_Val_read,IfVeSMSuSecRwLtStLgrstUpwdDnwdPosV_Val_read,IfVeSMSuSecRwLtStLtwdRtwdPosV_Val_read,IfVeSMSuSecRwLtStArmScrnPosV_Val_read
  Bus Selector5 : BusSelector  OutputSignals=IfVeSMSuSecRwLtStLgrstOtwdInwdPos_Val_read,IfVeSMSuRrLtStFtUpwdDnwdPos_Val_read,IfVeSMSuSecRwLtStHdrstFrwdBkwdPos_Val_read
  Bus Selector6 : BusSelector  OutputSignals=IfVeSMSuSecRwLtStLgrstOtwdInwdPosV_Val_read,IfVeSMSuRrLtStFtUpwdDnwdPosV_Val_read
  Bus Selector7 : BusSelector  OutputSignals=VipLSecRwLtSt.HdrstFrwdBkwdnwdPos,VipLSecRwLtSt.HdrstUpwdPos
  Chart : Stateflow chart  TreatAsAtomicUnit=on
  Chart1 : Stateflow chart  TreatAsAtomicUnit=on
  Logical Operator : Logic  Inputs=4  AllPortsSameDT=off  OutDataTypeStr=boolean
  Logical Operator1 : Logic  Inputs=3  AllPortsSameDT=off  OutDataTypeStr=boolean
  Logical Operator2 : Logic  AllPortsSameDT=off  OutDataTypeStr=boolean
  Logical Operator3 : Logic  AllPortsSameDT=off  OutDataTypeStr=boolean
  Logical Operator4 : Logic  Operator=NOT  AllPortsSameDT=off  OutDataTypeStr=boolean
  Logical Operator5 : Logic  AllPortsSameDT=off  OutDataTypeStr=boolean
  Logical Operator{6..9} (4 alike) : Logic  Operator=OR  AllPortsSameDT=off  OutDataTypeStr=boolean
  PA_KeSMSw4SSecRwLtStLgrstUpwdDnwdOpenPos1_Val : Constant  Value=KeSMSw4SSecRwLtStLgrstUpwdDnwdOpenPos1_Val
  R2Lt : Subsystem
  Relational Operator : RelationalOperator  OutDataTypeStr=boolean  RndMeth=Simplest
  Relational Operator1 : RelationalOperator  Operator=<  OutDataTypeStr=boolean  RndMeth=Simplest
  Relational Operator2 : RelationalOperator  Operator=<  OutDataTypeStr=boolean  RndMeth=Simplest
  Unit Delay1 : UnitDelay  SampleTime=-1
  Unit Delay3 : UnitDelay  SampleTime=-1
  Unit Delay4 : UnitDelay  SampleTime=-1
  VIP_TrigJudg : Lib/VIP_TrigJudg  SystemSampleTime=-1
  R2Lt_TrgtPoss : Outport  VectorParamsAs1DForOutWhenUnconnected=on
  IfVeSMSuSecRwLtStRclCmdSrv_Val_writeRec : Outport  Port=2
  isAcsMdFeedBackNew_LyL : Outport  Port=3
  R2Lt_TrgtPoss_2 : Outport  Port=4  VectorParamsAs1DForOutWhenUnconnected=on
  wires:
  Unit Delay4/1 -> Logical Operator3/2
  Logical Operator3/1 -> Chart/7(Step3done), [lgrstStep3_Chk]
  [lgrstStep2_Chk] -> Unit Delay4/1
  Unit Delay3/1 -> Logical Operator2/1
  R2Lt/11(R2Lt_TrgtPoss_2) -> R2Lt_TrgtPoss_2/1
  Unit Delay1/1 -> Chart/6(Step2done), [lgrstStep2_Chk]
  [lgrstStep2_done] -> Logical Operator2/2
  Relational Operator/1 -> Unit Delay3/1
  [OpenPos1] -> Relational Operator/2
  [SecRwLtStLgrstUpwdDnwdPos] -> Relational Operator/1
  [lgrstStep3_done] -> Logical Operator3/1
  Logical Operator2/1 -> Unit Delay1/1
  [OpenPos1] -> Chart/4(openpos1)
  PA_KeSMSw4SSecRwLtStLgrstUpwdDnwdOpenPos1_Val/1 -> [OpenPos1]
  [lgrstStep3_ini] -> Chart/10(Step3_ini)
  [lgrstStep2_ini] -> Chart/9(Step2_ini)
  [lgrstStep1_ini] -> Chart/8(Step1_ini)
  [lgrstStep1_done] -> Chart/5(Step1done)
  R2Lt/9(lgrstStep2_done) -> [lgrstStep2_done]
  R2Lt/10(lgrstStep3_done) -> [lgrstStep3_done]
  R2Lt/8(lgrstStep1_done) -> [lgrstStep1_done]
  R2Lt/6(lgrstStep2_ini) -> [lgrstStep2_ini]
  R2Lt/7(lgrstStep3_ini) -> [lgrstStep3_ini]
  R2Lt/5(lgrstStep1_ini) -> [lgrstStep1_ini]
  [StepEn_LgrstStep3] -> R2Lt/13(StepEn_LgrstStep3)
  [StepEn_LgrstStep2] -> R2Lt/12(StepEn_LgrstStep2)
  [StepEn_LgrstStep1] -> R2Lt/11(StepEn_LgrstStep1)
  [SecRwLtStLgrstUpwdDnwdPos] -> Chart/3(pos)
  Bus Selector5/2 -> [RrLtStFtUpwdDnwdPos]  "<IfVeSMSuRrLtStFtUpwdDnwdPos_Val_read>"
  Bus Selector5/1 -> [SecRwLtStLgrstOtwdInwdPos]  "<IfVeSMSuSecRwLtStLgrstOtwdInwdPos_Val_read>"
  [PosV4s] -> Bus Selector6/1
  Bus Selector6/2 -> [RrLtStFtUpwdDnwdPosV]  "<IfVeSMSuRrLtStFtUpwdDnwdPosV_Val_read>"
  [Pos4s] -> Bus Selector5/1
  Bus Selector6/1 -> [SecRwLtStLgrstOtwdInwdPosV]  "<IfVeSMSuSecRwLtStLgrstOtwdInwdPosV_Val_read>"
  Bus Selector4/1 -> [SecRwLtStBkReclnUpwdDnwdPosV]  "<IfVeSMSuSecRwLtStBkReclnUpwdDnwdPosV_Val_read>"
  Bus Selector4/3 -> [SecRwLtStHPassStUpwdDnwdPosV]  "<IfVeSMSuSecRwLtStHPassStUpwdDnwdPosV_Val_read>"
  Bus Selector3/5 -> [SecRwLtStLtwdRtwdPos]  "<IfVeSMSuSecRwLtStLtwdRtwdPos_Val_read>"
  [Pos] -> Bus Selector3/1
  Bus Selector3/3 -> [SecRwLtStHPassStUpwdDnwdPos]  "<IfVeSMSuSecRwLtStHPassStUpwdDnwdPos_Val_read>"
  Bus Selector4/4 -> [SecRwLtStLgrstUpwdDnwdPosV]  "<IfVeSMSuSecRwLtStLgrstUpwdDnwdPosV_Val_read>"
  Bus Selector4/2 -> [SecRwLtStFrwdBkwdPosV]  "<IfVeSMSuSecRwLtStFrwdBkwdPosV_Val_read>"
  Bus Selector3/2 -> [SecRwLtStFrwdBkwdPos]  "<IfVeSMSuSecRwLtStFrwdBkwdPos_Val_read>"
  Bus Selector3/1 -> [SecRwLtStBkReclnUpwdDnwdPos]  "<IfVeSMSuSecRwLtStBkReclnUpwdDnwdPos_Val_read>"
  Bus Selector3/4 -> [SecRwLtStLgrstUpwdDnwdPos]  "<IfVeSMSuSecRwLtStLgrstUpwdDnwdPos_Val_read>"
  Bus Selector4/5 -> [SecRwLtStLtwdRtwdPosV]  "<IfVeSMSuSecRwLtStLtwdRtwdPosV_Val_read>"
  Bus Selector3/6 -> [R2LtStArmScrnPos]  "<IfVeSMSuSecRwLtStArmScrnPos_Val_read>"
  Bus Selector4/6 -> [R2LtStArmScrnPosV]  "<IfVeSMSuSecRwLtStArmScrnPosV_Val_read>"
  [PosV] -> Bus Selector4/1
  [SecRwLtStConfig4s] -> R2Lt/10(StConfig4s)
  Bus Selector2/2 -> [SecRwRtStConfig4s]  "<SecRwRtStConfig>"
  Bus Selector2/1 -> [SecRwLtStConfig4s]  "<SecRwLtStConfig>"
  StConfig4s/1 -> Bus Selector2/1
  SecRwLtStPossV4s/1 -> R2Lt/9(SecRwLtStPossV4s), [PosV4s]
  SecRwLtStsPoss4s/1 -> R2Lt/8(SecRwLtStsPoss4s), [Pos4s]
  Bus Selector/7 -> [ModeStCalib_2L4s]  "<Calib_2L4s>"
  Bus Selector/8 -> [ModeStCalib_2R4s]  "<Calib_2R4s>"
  [SecRwLtStConfig] -> R2Lt/7(StConfig)
  Bus Selector1/5 -> [ThdRwLtStConfig]  "<ThdRwLtStConfig>"
  Bus Selector1/2 -> [PassStConfig]  "<PassStConfig>"
  StConfig/1 -> Bus Selector1/1
  Bus Selector1/4 -> [SecRwRtStConfig]  "<SecRwRtStConfig>"
  Bus Selector1/3 -> [SecRwLtStConfig]  "<SecRwLtStConfig>"
  Bus Selector1/1 -> [DrvStConfig]  "<DrvStConfig>"
  Bus Selector1/6 -> [ThdRwRtStConfig]  "<ThdRwRtStConfig>"
  [Ly_L_DoneFailed] -> Bus Creator1/2  "isLfVipDoneFailed"
  [Ly_L_DoneOK] -> Bus Creator1/1  "isLfVipDoneOK"
  Bus Creator1/1 -> isAcsMdFeedBackNew_LyL/1
  [Recovery_Mod_Left] -> VIP_TrigJudg/1
  [ModeStCalib_2L4s] -> R2Lt/6(ModeStCalib_2L)
  ModeStCalib/1 -> Bus Selector/1
  Bus Selector/4 -> [ModeStCalib_2R]  "<Calib_2R>"
  Bus Selector/6 -> [ModeStCalib_3R]  "<Calib_3R>"
  Bus Selector/1 -> [ModeStCalib_Drv]  "<Calib_Drv>"
  Bus Selector/3 -> [ModeStCalib_2L]  "<Calib_2L>"
  Bus Selector/5 -> [ModeStCalib_3L]  "<Calib_3L>"
  Bus Selector/2 -> [ModeStCalib_Pass]  "<Calib_Pass>"
  Chart1/1(IfVeSMSuSecRwLtStRclCmdSrv_Val_write) -> IfVeSMSuSecRwLtStRclCmdSrv_Val_writeRec/1  "IfVeSMSuSecRwLtStRclCmdSrv_Val_write"
  Chart1/3(Md_L_DoneFailed) -> [Ly_L_DoneFailed]
  Chart1/2(Md_L_DoneOk) -> [Ly_L_DoneOK]
  [Recv_L_DoneFailed] -> Chart1/4(Md_L_DoneFailedRaw)
  [Recv_L_DoneOK] -> Chart1/3(Md_L_DoneOkRaw)
  [R2LtST_BkHd_done] -> Chart/2(R2Lt_done)
  [R2LtST_BkHd_ini] -> Chart/1(R2Lt_ini)
  R2Lt/2(R2Lt_Bk_done) -> [R2LtST_BkHd_done]
  SecRwRtStChldLkRsp_L/1 -> R2Lt/5(SecRwRtStChldLkRsp_L)
  SecRwLtStPossV/1 -> R2Lt/4(SecRwLtStPossV), [PosV]
  SecRwLtStsPoss/1 -> R2Lt/3(SecRwLtStsPoss), [Pos]
  R2Lt/3(R2Lt_TrgtPoss) -> R2Lt_TrgtPoss/1
  [EZE_TrigL] -> R2Lt/1(Mode_Trig)
  VIP_TrigJudg/1 -> [EZE_TrigL]
  [Step1_En] -> R2Lt/2(Step1En)
  R2Lt/1(R2Lt_Bk_Ini) -> [R2LtST_BkHd_ini]
  Recovery_Mod_Left/1 -> [Recovery_Mod_Left]
  [IfVeSMSuSecRwLtStRclCmdSrv_Val_writeRaw] -> Chart1/2(IfVeSMSuSecRwLtStRclCmdSrv_Val_writeRaw)
  R2Lt/4(IfVeSMSuSecRwLtStRclCmdSrv_Val_writeRaw) -> [IfVeSMSuSecRwLtStRclCmdSrv_Val_writeRaw]
  Logical Operator4/1 -> [Recv_L_DoneFailed]
  isLfVipArrivedAtTargetPos/1 -> [Recv_L_DoneOK], Logical Operator4/1
  R2Lt/13(R2Lt_HdUp_Done) -> [HdUp_Done]
  R2Lt/15(R2Lt_HdFwd_Done) -> [HFwd_Done]
  R2Lt/12(R2Lt_HdUp_Ini) -> [HdUp_ini]
  R2Lt/14(R2Lt_HdFwd_Ini) -> [HFwd_ini]
  [HdUp_En] -> R2Lt/14(HdUp_En)
  [HdFwd_En] -> R2Lt/15(HdFwd_En)
  Chart/1(R2Lt_En) -> [Step1_En]
  [HdUp_Done] -> Chart/12(HdUp_Done)
  Chart/7(failflg) -> [failflg]
  Chart/5(HdUp_En) -> [HdUp_En]
  [HFwd_Done] -> Chart/13(HdFwd_Done)
  Chart/2(StepEn_LgrstStep1) -> [StepEn_LgrstStep1]
  Bus Selector7/1 -> Relational Operator1/2  "<HdrstFrwdBkwdnwdPos>"
  [SecRwLtStHdrstFrwdBkwdPos] -> Relational Operator1/1
  Logical Operator5/1 -> Chart/11(chkhdflg)
  Chart/6(HdFwd_En) -> [HdFwd_En]
  Relational Operator1/1 -> Logical Operator5/1
  [ModeStCalib_2L4s] -> Bus Selector7/1
  [SecRwLtStHPassStUpwdDnwdPos] -> Relational Operator2/1
  Bus Selector7/2 -> Relational Operator2/2  "<HdrstUpwdPos>"
  Chart/4(StepEn_LgrstStep3) -> [StepEn_LgrstStep3]
  Relational Operator2/1 -> Logical Operator5/2
  Chart/3(StepEn_LgrstStep2) -> [StepEn_LgrstStep2]
  [HdUp_Done] -> Logical Operator/3
  [HFwd_Done] -> Logical Operator/4
  [failflg] -> Logical Operator6/2
  Logical Operator1/1 -> Logical Operator6/1
  [R2LtST_BkHd_done] -> Logical Operator/2
  Logical Operator/1 -> Chart1/1(Left_Done)
  Logical Operator6/1 -> Logical Operator/1
  Bus Selector5/3 -> [SecRwLtStHdrstFrwdBkwdPos]  "<IfVeSMSuSecRwLtStHdrstFrwdBkwdPos_Val_read>"
  Logical Operator9/1 -> Logical Operator1/3
  Logical Operator8/1 -> Logical Operator1/2
  Logical Operator7/1 -> Logical Operator1/1
  [lgrstStep1_done] -> Logical Operator7/1
  [lgrstStep2_Chk] -> Logical Operator8/1
  [lgrstStep3_Chk] -> Logical Operator9/1
  [lgrstStep1_ini] -> Logical Operator7/2
  [lgrstStep2_ini] -> Logical Operator8/2
  [lgrstStep3_ini] -> Logical Operator9/2
  [HdUp_ini] -> Chart/14(HdUp_ini)
  [HFwd_ini] -> Chart/15(HdFwd_ini)
  Calib_VIP4sLAdpt/1 -> R2Lt/16(Calib_VIP4sLAdpt)

== system ModeAdjust/ModeAdjustRunnable_sys/ModeAdjust/VIPR ==
  SecRwRtStPoss : Inport
  SecRwRtStPossV : Inport  Port=2
  ThdRwRtStPoss : Inport  Port=3
  ThdRwRtStPossV : Inport  Port=4
  SecRwRtStChldLkRsp_R : Inport  Port=5
  isR3RtSeatOccupied : Inport  Port=6
  VIP_Mod_Right : Inport  Port=7
  ModeStCalib : Inport  Port=8
  is6s : Inport  Port=9
  ThdRwLtStPoss : Inport  Port=10
  ThdRwLtStPossV : Inport  Port=11
  isR3MidSeatOccupied : Inport  Port=12
  isR3LfSeatOccupied : Inport  Port=13
  StConfig : Inport  Port=14
  PassStPoss : Inport  Port=15
  PassStPossV : Inport  Port=16
  isRtVipArrivedAtTargetPos : Inport  Port=17
  PassSt_FtUpwdDnwdPosTrgt : Inport  Port=18
  Enable : EnablePort  StatesWhenEnabling=reset
  Bus Creator2 : BusCreator  Inputs=2
  Bus Selector : BusSelector  OutputSignals=Calib_Drv,Calib_Pass,Calib_2L,Calib_2R,Calib_3L,Calib_3R
  Bus Selector1 : BusSelector  OutputSignals=DrvStConfig,PassStConfig,SecRwLtStConfig,SecRwRtStConfig,ThdRwLtStConfig,ThdRwRtStConfig
  Chart1 : Stateflow chart  TreatAsAtomicUnit=on
  Chart2 : Stateflow chart  TreatAsAtomicUnit=on
  Logical Operator : Logic  Inputs=4  AllPortsSameDT=off  OutDataTypeStr=boolean
  Logical Operator1 : Logic  Operator=OR  AllPortsSameDT=off  OutDataTypeStr=boolean
  Logical Operator10 : Logic  Operator=OR  AllPortsSameDT=off  OutDataTypeStr=boolean
  Logical Operator{7,12,14..15} (4 alike) : Logic  AllPortsSameDT=off  OutDataTypeStr=boolean
  Logical Operator13 : Logic  Inputs=3  AllPortsSameDT=off  OutDataTypeStr=boolean
  Logical Operator2 : Logic  Operator=NOT  AllPortsSameDT=off  OutDataTypeStr=boolean
  Logical Operator4 : Logic  Operator=OR  Inputs=3  AllPortsSameDT=off  OutDataTypeStr=boolean
  Logical Operator5 : Logic  Inputs=4  AllPortsSameDT=off  OutDataTypeStr=boolean
  Logical Operator6 : Logic  Inputs=3  AllPortsSameDT=off  OutDataTypeStr=boolean
  Logical Operator8 : Logic  Operator=OR  AllPortsSameDT=off  OutDataTypeStr=boolean
  PA_KeSMSwDltTrgtPos_Val5 : Constant  Value=0  OutDataTypeStr=boolean
  Pass : Subsystem
  R2Rt : Subsystem
  R3Lt : Subsystem
  R3Rt : Subsystem
  Switch : Switch  Criteria=u2 > Threshold
  Terminator4 : Terminator
  Unit Delay : UnitDelay  SampleTime=-1
  Unit Delay3 : UnitDelay  SampleTime=-1
  Unit Delay4 : UnitDelay  SampleTime=-1
  VIP_TrigJudg1 : Lib/VIP_TrigJudg  SystemSampleTime=-1
  R2Rt_TrgtPoss : Outport  VectorParamsAs1DForOutWhenUnconnected=on
  R3Rt_TrgtPoss : Outport  Port=2  VectorParamsAs1DForOutWhenUnconnected=on
  IfVeSMSbThdRwRtStRclCmdSrv_Val_writeVIP : Outport  Port=3
  IfVeSMSbSecRwRtStRclCmdSrv_Val_writeVIP : Outport  Port=4
  isAcsMdFeedBackNew_VIPR : Outport  Port=5
  VIPRDone : Outport  Port=6
  R3Lt_TrgtPoss : Outport  Port=7  VectorParamsAs1DForOutWhenUnconnected=on
  IfVeSMSbThdRwLtStRclCmdSrv_Val_writeVIP : Outport  Port=8
  PassStTrgtPoss : Outport  Port=9  VectorParamsAs1DForOutWhenUnconnected=on
  IfVeSMSuPassStRclCmdSrv_Val_writeVIP : Outport  Port=10
  R2Rt_SpdCtrl : Outport  Port=11  VectorParamsAs1DForOutWhenUnconnected=on
  R3Rt_SpdCtrl : Outport  Port=12  VectorParamsAs1DForOutWhenUnconnected=on
  R3Lt_SpdCtrl : Outport  Port=13  VectorParamsAs1DForOutWhenUnconnected=on
  wires:
  Bus Creator2/1 -> isAcsMdFeedBackNew_VIPR/1
  [VIP_R_DoneOK] -> Bus Creator2/1  "isRtVipDoneOK"
  [VIP_R_DoneFailed] -> Bus Creator2/2  "isRtVipDoneFailed"
  VIP_TrigJudg1/1 -> [EZE_TrigR]
  [VIP_right] -> VIP_TrigJudg1/1
  Logical Operator13/1 -> VIPRDone/1, Chart1/1(RightDone)
  is6s/1 -> [is6s]
  [ModeStCalib_3R] -> R3Rt/6(ModeStCalib_3R)
  [ModeStCalib_2R] -> R2Rt/8(ModeStCalib_2R)
  ModeStCalib/1 -> Bus Selector/1
  Bus Selector/4 -> [ModeStCalib_2R]  "<Calib_2R>"
  Bus Selector/6 -> [ModeStCalib_3R]  "<Calib_3R>"
  Bus Selector/1 -> [ModeStCalib_Drv]  "<Calib_Drv>"
  Bus Selector/3 -> [ModeStCalib_2L]  "<Calib_2L>"
  Bus Selector/5 -> [ModeStCalib_3L]  "<Calib_3L>"
  Bus Selector/2 -> [ModeStCalib_Pass]  "<Calib_Pass>"
  R3Rt/5(R3Rt_All_done) -> [R3Rt_All_done]
  R2Rt/11(R2Rt_All_done) -> [R2RtST_All_done]
  Chart1/2(IfVeSMSbSecRwRtStRclCmdSrv_Val_write) -> IfVeSMSbSecRwRtStRclCmdSrv_Val_writeVIP/1  "IfVeSMSbSecRwRtStRclCmdSrv_Val_write"
  Chart1/1(IfVeSMSbThdRwRtStRclCmdSrv_Val_write) -> IfVeSMSbThdRwRtStRclCmdSrv_Val_writeVIP/1  "IfVeSMSbThdRwRtStRclCmdSrv_Val_write"
  Chart1/4(Md_R_DoneFailed) -> [VIP_R_DoneFailed]
  Chart1/3(Md_R_DoneOk) -> [VIP_R_DoneOK]
  [Md_R_MvDoneFailed] -> Chart1/5(Md_R_DoneFailedRaw)
  [Md_R_MvDoneOK] -> Chart1/4(Md_R_DoneOkRaw)
  R2Rt/10(IfVeSMSbSecRwRtStRclCmdSrv_Val_writeRaw) -> [IfVeSMSbSecRwRtStRclCmdSrv_Val_writeRaw]
  [IfVeSMSbSecRwRtStRclCmdSrv_Val_writeRaw] -> Chart1/3(IfVeSMSbSecRwRtStRclCmdSrv_Val_writeRaw)
  VIP_Mod_Right/1 -> [VIP_right]
  [R3Lt_Step1_done] -> Chart2/6(L_R3Step1done)
  [R3Lt_Step1_ini] -> Chart2/1(L_R3Step1_ini)
  [R3Lt_Step1_ini] -> [L_R3_ini]
  [R_R2Step3] -> R2Rt/4(Step3En)
  [R_R2Step2] -> R2Rt/3(Step2En)
  [R_R2Step1] -> R2Rt/2(Step1En)
  [R_R3Step1] -> R3Rt/2(Step1En)
  Chart2/1(R_R3Step1) -> [R_R3Step1]
  [R2RtST_Step2_done] -> Chart2/8(L_R2Step2done)
  [R2RtST_Step1_done] -> Chart2/7(L_R2Step1done)
  [R_ini_ReclnOverUp] -> Chart2/5(L_PosOvrup)
  [R3Rt_Step1_done] -> Chart2/10(R_R3Step1done)
  [R3Rt_Step1_ini] -> Chart2/9(R_R3Step1_ini)
  [R3Rt_Step1_ini] -> [R_R3_ini_done]
  [R2RtST_Step2_ini] -> Chart2/3(L_R2Step2_ini)
  [R2RtST_Step1_ini] -> Chart2/2(L_R2Step1_ini)
  Logical Operator6/1 -> [R_R2_ini]
  [R2RtST_Step3_ini] -> Logical Operator6/3
  [R2RtST_Step2_ini] -> Logical Operator6/2
  [R2RtST_Step1_ini] -> Logical Operator6/1
  [R2RtST_Step3_ini] -> Chart2/4(L_R2Step3_ini)
  R2Rt/9(R2Rt_Step3_done) -> [R2RtST_Step3_done]  "VIPR_R2RtST_Step3_done"
  R2Rt/8(R2RtSt_Step3_ini) -> [R2RtST_Step3_ini]
  R2Rt/3(ini_ReclnOverDwn) -> Terminator4/1
  R2Rt/2(ini_ReclnOverUp) -> [R_ini_ReclnOverUp]
  [EZE_TrigR] -> R3Rt/1(Mode_Trig)
  R3Rt/1(R3Rt_Step1_ini) -> [R3Rt_Step1_ini]
  R2Rt/1(R2RtSt_Step1_ini) -> [R2RtST_Step1_ini]
  R2Rt/4(R2RtSt_Step2_ini) -> [R2RtST_Step2_ini]
  R2Rt/5(R2Rt_Step1_done) -> [R2RtST_Step1_done]  "VIPR_R2RtST_Step1_done"
  R2Rt/6(R2Rt_Step2_done) -> [R2RtST_Step2_done]  "VIPR_R2RtST_Step2_done"
  R3Rt/2(R3Rt__Step1done) -> [R3Rt_Step1_done]  "VIPR_R3Rt_Step1_done"
  R3Rt/3(IfVeSMSbThdRwRtStRclCmdSrv_Val_writeRaw) -> [IfVeSMSbThdRwRtStRclCmdSrv_Val_writeRaw]
  [IfVeSMSbThdRwRtStRclCmdSrv_Val_writeRaw] -> Chart1/2(IfVeSMSbThdRwRtStRclCmdSrv_Val_writeRaw)
  [EZE_TrigR] -> R2Rt/1(Mode_Trig)
  R2Rt/7(R2Rt_TrgtPoss) -> R2Rt_TrgtPoss/1
  R3Rt/4(R3Rt_TrgtPoss) -> R3Rt_TrgtPoss/1
  ThdRwRtStPoss/1 -> R3Rt/4(ThdRwRtStPoss)
  ThdRwRtStPossV/1 -> R3Rt/5(ThdRwRtStPossV)
  SecRwRtStPoss/1 -> R2Rt/5(SecRwRtStPoss)
  SecRwRtStPossV/1 -> R2Rt/6(SecRwRtStPossV)
  SecRwRtStChldLkRsp_R/1 -> [SecRwRtStChldLkRsp_R], R2Rt/7(SecRwRtStChldLkRsp_L)
  [ModeStCalib_3L] -> R3Lt/6(ModeStCalib_3L)
  ThdRwLtStPossV/1 -> R3Lt/5(ThdRwLtStPossV)
  [is6s] -> R3Lt/7(is6s)
  R3Lt/5(R3Lt_All_done) -> [R3Lt_All_done]
  R3Lt/3(IfVeSMSbThdRwLtStRclCmdSrv_Val_writeRaw) -> [IfVeSMSbThdRwLtStRclCmdSrv_Val_writeRaw]
  [L_R3Step1] -> R3Lt/2(Step1En)
  R3Lt/1(R3Lt_Step1_ini) -> [R3Lt_Step1_ini]
  R3Lt/2(R3Lt_Step1done) -> [R3Lt_Step1_done]  "VIPR_R3Lt_Step1_done"
  R3Lt/4(R3Lt_TrgtPoss) -> R3Lt_TrgtPoss/1
  ThdRwLtStPoss/1 -> R3Lt/4(ThdRwLtStPoss)
  [EZE_TrigR] -> R3Lt/1(Mode_Trig)
  isR3MidSeatOccupied/1 -> Logical Operator4/2
  [IfVeSMSbThdRwLtStRclCmdSrv_Val_writeRaw] -> Chart1/6(IfVeSMSbThdRwLtStRclCmdSrv_Val_writeRaw)
  Chart1/5(IfVeSMSbThdRwLtStRclCmdSrv_Val_write) -> IfVeSMSbThdRwLtStRclCmdSrv_Val_writeVIP/1
  Bus Selector1/6 -> [ThdRwRtStConfig]  "<ThdRwRtStConfig>"
  Bus Selector1/1 -> [DrvStConfig]  "<DrvStConfig>"
  Bus Selector1/3 -> [SecRwLtStConfig]  "<SecRwLtStConfig>"
  Bus Selector1/4 -> [SecRwRtStConfig]  "<SecRwRtStConfig>"
  StConfig/1 -> Bus Selector1/1
  Bus Selector1/2 -> [PassStConfig]  "<PassStConfig>"
  Bus Selector1/5 -> [ThdRwLtStConfig]  "<ThdRwLtStConfig>"
  [ThdRwLtStConfig] -> R3Lt/8(StConfig)
  [ThdRwRtStConfig] -> R3Rt/7(StConfig)
  [SecRwRtStConfig] -> R2Rt/9(StConfig)
  isR3RtSeatOccupied/1 -> Logical Operator4/3
  Logical Operator4/1 -> [Occupied]
  [Occupied] -> R3Lt/3(isSeatOccupied)
  [Occupied] -> R3Rt/3(SeatOccupied)
  [Occupied] -> R2Rt/10(isSeatOccupied)
  [SecRwRtStChldLkRsp_R] -> R3Lt/9(SecRwRtStChldLkRsp_L)
  [SecRwRtStChldLkRsp_R] -> R3Rt/8(SecRwRtStChldLkRsp_L)
  [is6s] -> Switch/2
  Switch/1 -> Logical Operator4/1
  Pass/2(Pass_Step1_done) -> [Pass_Step1_done]  "VIPR_Pass_Step1_done"
  [EZE_TrigR] -> Pass/1(Mode_Trig)
  Pass/4(IfVeSMSuPassStRclCmdSrv_Val_writeRaw) -> [IfVeSMSuPassStRclCmdSrv_Val_writeRaw]
  PassStPossV/1 -> Pass/4(PassStPossV)
  [PassStConfig] -> Pass/6(StConfig)
  Pass/1(Pass_Step1_ini) -> [PassST_Step1_ini]
  Pass/3(PassStTrgtPoss) -> PassStTrgtPoss/1
  [ModeStCalib_Pass] -> Pass/5(ModeStCalib_Pass)
  [R_R1Step1] -> Pass/2(Step1En)
  PassStPoss/1 -> Pass/3(PassStPoss)
  Chart2/2(L_R3Step1) -> [L_R3Step1]
  Chart2/3(L_R2Step1) -> [R_R2Step1]
  Chart2/4(L_R2Step2) -> [R_R2Step2]
  Chart2/5(L_R2Step3) -> [R_R2Step3]
  Chart2/6(L_R1Step1) -> [R_R1Step1]
  [PassST_Step1_ini] -> Chart2/13(L_R1Step1_ini)
  [R3Rt_Step1_done] -> Logical Operator/2
  [R2RtST_Step2_done] -> Logical Operator/4
  [R3Lt_Step1_done] -> Logical Operator/1
  [R2RtST_Step1_done] -> Logical Operator/3
  [Stage1_done] -> Chart2/11(Stage1_done)
  [Stage2_done] -> Chart2/12(Stage2_done)
  [IfVeSMSuPassStRclCmdSrv_Val_writeRaw] -> Chart1/7(IfVeSMSuPassStRclCmdSrv_Val_writeRaw)
  Chart1/6(IfVeSMSuPassStRclCmdSrv_Val_write) -> IfVeSMSuPassStRclCmdSrv_Val_writeVIP/1
  Logical Operator/1 -> Unit Delay/1
  Logical Operator1/1 -> [Stage1_done]
  Unit Delay/1 -> Logical Operator1/2
  [R2RtST_Step1_ini] -> Logical Operator5/1
  [R2RtST_Step2_ini] -> Logical Operator5/2
  [R_R3_ini_done] -> Logical Operator5/3
  [L_R3_ini] -> Logical Operator5/4
  Logical Operator5/1 -> Logical Operator1/1
  [Pass_Step1_done] -> Logical Operator7/1
  [Stage1_done] -> Unit Delay3/1
  Logical Operator7/1 -> Logical Operator8/2
  Logical Operator8/1 -> [Stage2_done]
  [Stage2_done] -> Unit Delay4/1
  Logical Operator12/1 -> Logical Operator10/2
  Logical Operator10/1 -> [Stage3_done]
  [Stage1_done] -> Logical Operator13/1
  [Stage2_done] -> Logical Operator13/2
  [Stage3_done] -> Logical Operator13/3
  [R2RtST_Step3_done] -> Logical Operator12/1
  [Stage3_done] -> Chart2/14(Stage3_done)
  Unit Delay3/1 -> Logical Operator7/2
  Unit Delay4/1 -> Logical Operator12/2
  Logical Operator14/1 -> Logical Operator10/1
  [R2RtST_Step3_ini] -> Logical Operator14/1
  [Stage2_done] -> Logical Operator14/2
  [PassST_Step1_ini] -> Logical Operator15/1
  Logical Operator15/1 -> Logical Operator8/1
  [Stage1_done] -> Logical Operator15/2
  [SecRwRtStChldLkRsp_R] -> Pass/7(SecRwRtStChldLkRsp_L)
  [Occupied] -> Pass/8(isSeatOccupied)
  Logical Operator2/1 -> [Md_R_MvDoneFailed]
  isRtVipArrivedAtTargetPos/1 -> [Md_R_MvDoneOK], Logical Operator2/1
  PassSt_FtUpwdDnwdPosTrgt/1 -> Pass/9(PassSt_FtUpwdDnwdPosTrgt)
  R2Rt/12(R2Rt_SpdCtrl) -> R2Rt_SpdCtrl/1
  R3Rt/6(R3Rt_SpdCtrl) -> R3Rt_SpdCtrl/1
  R3Lt/6(R3Lt_SpdCtrl) -> R3Lt_SpdCtrl/1
  PA_KeSMSwDltTrgtPos_Val5/1 -> Switch/1
  isR3LfSeatOccupied/1 -> Switch/3
